simulink model "r2daq"  (R2012b)
settings: Solver=FixedStepDiscrete  SolverMode=SingleTasking  StartTime=0.0  StopTime=10.0  RelTol=1e-3
PreLoadFcn:
  | addpath(genpath('../lib/'));
model workspace (MAT data in the model file):
  pd_coeffbanks = 4
  pd_synthconf = 4
  pd_ctrl_reg = 4
  pd_ddc_2nd_stage = 64
  pd_status_reg = 4
  delay_time_pkt_vs_freq_pkt = 1536
  pd_to_status = 16
  pd_quantize = 16
undefined symbols (not defined in the file or in its folder): sfp
libraries: xbsIndex_r4 x1116, filters x8, r2daq_blocks x7, casper_library_misc x6, xps_library x3, synths x1, simulink x1
(part 1 of 14)
settings Model: Creator=ayoung  LastModifiedBy=ayoung
settings DebuggingCC: SigSpecEnsureSampleTimeMsg=none

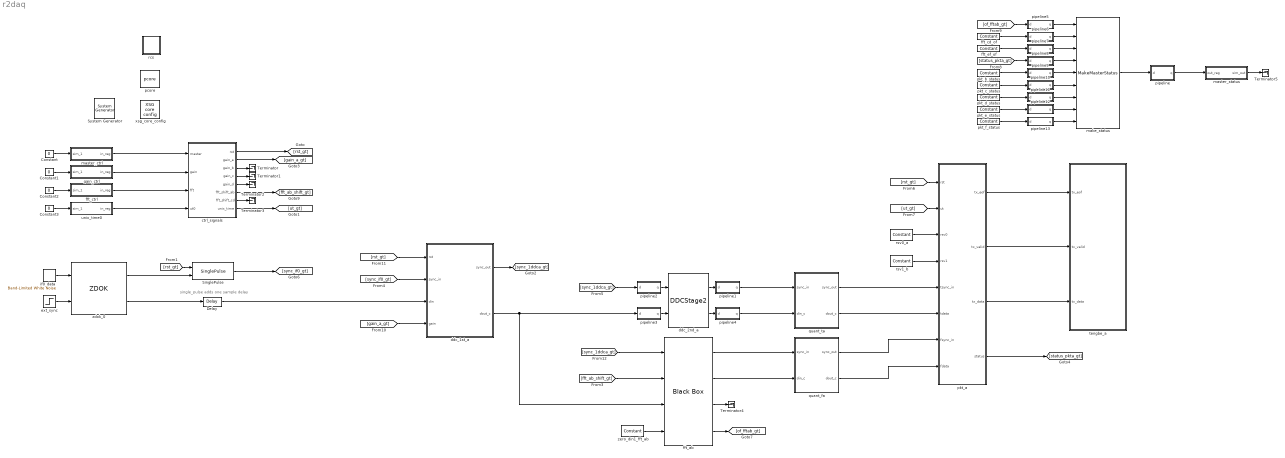
== system r2daq ==
  note: single_pulse adds one sample delay
  " System Generator" : xbsIndex_r4/ System Generator  Tag=genX  xilinxfamily=virtex6  part=xc6vsx475t  speed=-1  package=ff1759  synthesis_tool=XST  clock_wrapper=Clock Enables  directory=./r2daq/sysgen  proj_type=Project Navigator  Synth_file=XST Defaults  Impl_file=ISE Defaults  testbench=off  simulink_period=1  sysclk_period=5  dcm_input_clock_period=100  incr_netlist=off  trim_vbits=Everywhere in SubSystem  dbl_ovrd=According to Block Masks  core_generation=According to Block Masks  run_coregen=off  deprecated_control=off  eval_field=0  block_type=sysgen
  Constant{,1..3} (4 alike) : Constant  Value=0
  Delay : xbsIndex_r4/Delay  rst=off  infoeditControl=Selection of Reset will increase slice count due to use of real FFs and instead of SRLs  en=off  latency=1  dbl_ovrd=off  reg_retiming=off  block_type=delay
  SinglePulse : r2daq_blocks/SinglePulse
  Terminator{,1..5} (6 alike) : Terminator
  ctrl_signals : Subsystem
  ddc_1st_a : Subsystem
  ddc_2nd_a : r2daq_blocks/DDCStage2
  ext_sync : Step  SampleTime=0
  fft_ab : xbsIndex_r4/Black Box  init_code=fft_core_config  sim_method=Inactive  verbose=off  block_type=blackbox2
  fft_cd_of : xbsIndex_r4/Constant  const=0  gui_display_data_type=Boolean  arith_type=Boolean  n_bits=4  bin_pt=0  preci_type=Single  exp_width=8  frac_width=24  explicit_period=on  period=1  equ=P=C  opselect=C  inp2=PCIN>>17  opr=+  inp1=P  carry=CIN  dbl_ovrd=off  block_type=constant
  fft_ctrl : Subsystem  Tag=xps:sw_reg  AncestorBlock=xps_library/software_register  mask(swreg){mode=one value, io_dir=From Processor, io_delay=0, sample_period=1, names=reg, bitwidths=32, arith_types=0, bin_pts=0, sim_port=on, show_format=off}
      mask prompts: io_dir "I/O direction"; io_delay "I/O delay"; sample_period "Sample period"; names "Name:"; bitwidths "Bitwidth:"; arith_types "Type (ufix=0, fix=1, bool=2):"; bin_pts "Binary pt:"; sim_port "Provide sim input/output?"; show_format "Print format string?"
      mask init:
      | swreg_init(gcb)
      settings: AttributesFormatString=1input
      mask TypeOptions mode: one value | fields of equal size | fields of arbitrary size
      mask Callback mode: swreg_cb(gcb);
      mask TypeOptions io_dir: To Processor | From Processor
      mask Callback io_dir:
      | mask_enables = get_param(gcb, 'MaskEnables');
      | mask_names = get_param(gcb, 'MaskNames');
      | if strcmp(get_param(gcb, 'io_dir'), 'To Processor'),
      |     mask_enables{ismember(mask_names, 'sample_period')} = 'off';
      | else
      |     mask_enables{ismember(mask_names, 'sample_period')} = 'on';
      | end
      | set_param(gcb, 'MaskEnables', mask_enables);
      mask Callback bitwidths:
      | swreg_maskcheck(gcb);
      | % blk = gcb;
      | % mode = get_param(blk, 'mode');
      | % current_widths = eval(get_param(blk, 'bitwidths'));
      | % if (strcmp(mode, 'one value') || strcmp(mode, 'fields of equal size')) && (length(current_widths) > 1),
      | %     error('Only one width may be specified for this mode.');
      | % elseif strcmp(mode, 'fields of arbitrary size')
      | %     current_names = textscan(strtrim(strrep(strrep(get_param(blk, 'names'), ']', ''), '[', '')), '%s');
      | %     current_names = current_names{1};
      | %     numios = length(current_names);
      | %     if length(current_widths) ~= numios,
      | %         error('%d field names specified, but %d widths?', numios, length(current_widths));
      | %     end
      | % end
      | % total_width = 0;
      | % for ctr = 1 : length(current_widths),
      | %     total_width = total_width + current_widths(ctr);
      | % end
      | % if total_width > 32,
      | %     error('Total width must be 32 or less, set to %d.', total_width);
      | % end
      mask Callback arith_types:
      | [numios, ~, ~, ~, current_types] = swreg_maskcheck(gcb);
      | % blk = gcb;
      | % mode = get_param(blk, 'mode');
      | % current_types = eval(get_param(blk, 'arith_types'));
      | % numios = length(current_types);
      | % if (strcmp(mode, 'one value') || strcmp(mode, 'fields of equal size')) && (length(current_types) > 1),
      | %     error('Only one type may be specified for this mode.');
      | % elseif strcmp(mode, 'fields of arbitrary size')
      | %     current_names = textscan(strtrim(strrep(strrep(get_param(blk, 'names'), ']', ''), '[', '')), '%s');
      | %     current_names = current_names{1};
      | %     numios = length(current_names);
      | %     if length(current_types) ~= numios,
      | %         error('%d field names specified, but %d types?', numios, length(current_types));
      | %     end
      | % end
      | problem = 0;
      | for ctr = 1 : numios,
      |     t = current_types(ctr);
      |     if (t < 0) || (t > 2),
      |         problem = t;
      |         ctr = numios + 1;
      |     end
      | end
      | if problem ~= 0,
      |     error('Type cannot be %i, must be 0, 1 or 2.', problem);
      | end
      mask Callback bin_pts:
      | swreg_maskcheck(gcb);
      | % blk = gcb;
      | % mode = get_param(blk, 'mode');
      | % current_bins = eval(get_param(blk, 'bin_pts'));
      | % if (strcmp(mode, 'one value') || strcmp(mode, 'fields of equal size')) && (length(current_bins) > 1),
      | %     error('Only one binary pt may be specified for this mode.');
      | % elseif strcmp(mode, 'fields of arbitrary size')
      | %     current_names = textscan(strtrim(strrep(strrep(get_param(blk, 'names'), ']', ''), '[', '')), '%s');
      | %     current_names = current_names{1};
      | %     numios = length(current_names);
      | %     if length(current_bins) ~= numios,
      | %         error('%d field names specified, but %d binary pts?', numios, length(current_bins));
      | %     end
      | % end
  fft_ef_of : xbsIndex_r4/Constant  const=0  gui_display_data_type=Boolean  arith_type=Boolean  n_bits=4  bin_pt=0  preci_type=Single  exp_width=8  frac_width=24  explicit_period=on  period=1  equ=P=C  opselect=C  inp2=PCIN>>17  opr=+  inp1=P  carry=CIN  dbl_ovrd=off  block_type=constant
  gain_ctrl : Subsystem  Tag=xps:sw_reg  AncestorBlock=xps_library/software_register  mask(swreg){mode=one value, io_dir=From Processor, io_delay=0, sample_period=1, names=reg, bitwidths=32, arith_types=0, bin_pts=0, sim_port=on, show_format=off}
      mask prompts: io_dir "I/O direction"; io_delay "I/O delay"; sample_period "Sample period"; names "Name:"; bitwidths "Bitwidth:"; arith_types "Type (ufix=0, fix=1, bool=2):"; bin_pts "Binary pt:"; sim_port "Provide sim input/output?"; show_format "Print format string?"
      mask init:
      | swreg_init(gcb)
      settings: AttributesFormatString=1input
      mask TypeOptions mode: one value | fields of equal size | fields of arbitrary size
      mask Callback mode: swreg_cb(gcb);
      mask TypeOptions io_dir: To Processor | From Processor
      mask Callback io_dir:
      | mask_enables = get_param(gcb, 'MaskEnables');
      | mask_names = get_param(gcb, 'MaskNames');
      | if strcmp(get_param(gcb, 'io_dir'), 'To Processor'),
      |     mask_enables{ismember(mask_names, 'sample_period')} = 'off';
      | else
      |     mask_enables{ismember(mask_names, 'sample_period')} = 'on';
      | end
      | set_param(gcb, 'MaskEnables', mask_enables);
      mask Callback bitwidths:
      | swreg_maskcheck(gcb);
      | % blk = gcb;
      | % mode = get_param(blk, 'mode');
      | % current_widths = eval(get_param(blk, 'bitwidths'));
      | % if (strcmp(mode, 'one value') || strcmp(mode, 'fields of equal size')) && (length(current_widths) > 1),
      | %     error('Only one width may be specified for this mode.');
      | % elseif strcmp(mode, 'fields of arbitrary size')
      | %     current_names = textscan(strtrim(strrep(strrep(get_param(blk, 'names'), ']', ''), '[', '')), '%s');
      | %     current_names = current_names{1};
      | %     numios = length(current_names);
      | %     if length(current_widths) ~= numios,
      | %         error('%d field names specified, but %d widths?', numios, length(current_widths));
      | %     end
      | % end
      | % total_width = 0;
      | % for ctr = 1 : length(current_widths),
      | %     total_width = total_width + current_widths(ctr);
      | % end
      | % if total_width > 32,
      | %     error('Total width must be 32 or less, set to %d.', total_width);
      | % end
      mask Callback arith_types:
      | [numios, ~, ~, ~, current_types] = swreg_maskcheck(gcb);
      | % blk = gcb;
      | % mode = get_param(blk, 'mode');
      | % current_types = eval(get_param(blk, 'arith_types'));
      | % numios = length(current_types);
      | % if (strcmp(mode, 'one value') || strcmp(mode, 'fields of equal size')) && (length(current_types) > 1),
      | %     error('Only one type may be specified for this mode.');
      | % elseif strcmp(mode, 'fields of arbitrary size')
      | %     current_names = textscan(strtrim(strrep(strrep(get_param(blk, 'names'), ']', ''), '[', '')), '%s');
      | %     current_names = current_names{1};
      | %     numios = length(current_names);
      | %     if length(current_types) ~= numios,
      | %         error('%d field names specified, but %d types?', numios, length(current_types));
      | %     end
      | % end
      | problem = 0;
      | for ctr = 1 : numios,
      |     t = current_types(ctr);
      |     if (t < 0) || (t > 2),
      |         problem = t;
      |         ctr = numios + 1;
      |     end
      | end
      | if problem ~= 0,
      |     error('Type cannot be %i, must be 0, 1 or 2.', problem);
      | end
      mask Callback bin_pts:
      | swreg_maskcheck(gcb);
      | % blk = gcb;
      | % mode = get_param(blk, 'mode');
      | % current_bins = eval(get_param(blk, 'bin_pts'));
      | % if (strcmp(mode, 'one value') || strcmp(mode, 'fields of equal size')) && (length(current_bins) > 1),
      | %     error('Only one binary pt may be specified for this mode.');
      | % elseif strcmp(mode, 'fields of arbitrary size')
      | %     current_names = textscan(strtrim(strrep(strrep(get_param(blk, 'names'), ']', ''), '[', '')), '%s');
      | %     current_names = current_names{1};
      | %     numios = length(current_names);
      | %     if length(current_bins) ~= numios,
      | %         error('%d field names specified, but %d binary pts?', numios, length(current_bins));
      | %     end
      | % end
  if0_data : simulink/Sources/Band-Limited White Noise  Cov=[0.1]  Ts=0.1  seed=[23341]
  make_status : r2daq_blocks/MakeMasterStatus
  master_ctrl : Subsystem  Tag=xps:sw_reg  AncestorBlock=xps_library/software_register  mask(swreg){mode=one value, io_dir=From Processor, io_delay=0, sample_period=1, names=reg, bitwidths=32, arith_types=0, bin_pts=0, sim_port=on, show_format=off}
      mask prompts: io_dir "I/O direction"; io_delay "I/O delay"; sample_period "Sample period"; names "Name:"; bitwidths "Bitwidth:"; arith_types "Type (ufix=0, fix=1, bool=2):"; bin_pts "Binary pt:"; sim_port "Provide sim input/output?"; show_format "Print format string?"
      mask init:
      | swreg_init(gcb)
      settings: AttributesFormatString=1input
      mask TypeOptions mode: one value | fields of equal size | fields of arbitrary size
      mask Callback mode: swreg_cb(gcb);
      mask TypeOptions io_dir: To Processor | From Processor
      mask Callback io_dir:
      | mask_enables = get_param(gcb, 'MaskEnables');
      | mask_names = get_param(gcb, 'MaskNames');
      | if strcmp(get_param(gcb, 'io_dir'), 'To Processor'),
      |     mask_enables{ismember(mask_names, 'sample_period')} = 'off';
      | else
      |     mask_enables{ismember(mask_names, 'sample_period')} = 'on';
      | end
      | set_param(gcb, 'MaskEnables', mask_enables);
      mask Callback bitwidths:
      | swreg_maskcheck(gcb);
      | % blk = gcb;
      | % mode = get_param(blk, 'mode');
      | % current_widths = eval(get_param(blk, 'bitwidths'));
      | % if (strcmp(mode, 'one value') || strcmp(mode, 'fields of equal size')) && (length(current_widths) > 1),
      | %     error('Only one width may be specified for this mode.');
      | % elseif strcmp(mode, 'fields of arbitrary size')
      | %     current_names = textscan(strtrim(strrep(strrep(get_param(blk, 'names'), ']', ''), '[', '')), '%s');
      | %     current_names = current_names{1};
      | %     numios = length(current_names);
      | %     if length(current_widths) ~= numios,
      | %         error('%d field names specified, but %d widths?', numios, length(current_widths));
      | %     end
      | % end
      | % total_width = 0;
      | % for ctr = 1 : length(current_widths),
      | %     total_width = total_width + current_widths(ctr);
      | % end
      | % if total_width > 32,
      | %     error('Total width must be 32 or less, set to %d.', total_width);
      | % end
      mask Callback arith_types:
      | [numios, ~, ~, ~, current_types] = swreg_maskcheck(gcb);
      | % blk = gcb;
      | % mode = get_param(blk, 'mode');
      | % current_types = eval(get_param(blk, 'arith_types'));
      | % numios = length(current_types);
      | % if (strcmp(mode, 'one value') || strcmp(mode, 'fields of equal size')) && (length(current_types) > 1),
      | %     error('Only one type may be specified for this mode.');
      | % elseif strcmp(mode, 'fields of arbitrary size')
      | %     current_names = textscan(strtrim(strrep(strrep(get_param(blk, 'names'), ']', ''), '[', '')), '%s');
      | %     current_names = current_names{1};
      | %     numios = length(current_names);
      | %     if length(current_types) ~= numios,
      | %         error('%d field names specified, but %d types?', numios, length(current_types));
      | %     end
      | % end
      | problem = 0;
      | for ctr = 1 : numios,
      |     t = current_types(ctr);
      |     if (t < 0) || (t > 2),
      |         problem = t;
      |         ctr = numios + 1;
      |     end
      | end
      | if problem ~= 0,
      |     error('Type cannot be %i, must be 0, 1 or 2.', problem);
      | end
      mask Callback bin_pts:
      | swreg_maskcheck(gcb);
      | % blk = gcb;
      | % mode = get_param(blk, 'mode');
      | % current_bins = eval(get_param(blk, 'bin_pts'));
      | % if (strcmp(mode, 'one value') || strcmp(mode, 'fields of equal size')) && (length(current_bins) > 1),
      | %     error('Only one binary pt may be specified for this mode.');
      | % elseif strcmp(mode, 'fields of arbitrary size')
      | %     current_names = textscan(strtrim(strrep(strrep(get_param(blk, 'names'), ']', ''), '[', '')), '%s');
      | %     current_names = current_names{1};
      | %     numios = length(current_names);
      | %     if length(current_bins) ~= numios,
      | %         error('%d field names specified, but %d binary pts?', numios, length(current_bins));
      | %     end
      | % end
  master_status : Subsystem  Tag=xps:sw_reg  AncestorBlock=xps_library/software register  mask(swreg){mode=one value, io_dir=To Processor, io_delay=0, sample_period=1, names=reg, bitwidths=32, arith_types=0, bin_pts=0, sim_port=on, show_format=off}
      mask prompts: io_dir "I/O direction"; io_delay "I/O delay"; sample_period "Sample period"; names "Name:"; bitwidths "Bitwidth:"; arith_types "Type (ufix=0, fix=1, bool=2):"; bin_pts "Binary pt:"; sim_port "Provide sim input/output?"; show_format "Print format string?"
      mask init:
      | swreg_init(gcb)
      settings: AttributesFormatString=1output
      mask TypeOptions mode: one value | fields of equal size | fields of arbitrary size
      mask Callback mode: swreg_cb(gcb);
      mask TypeOptions io_dir: To Processor | From Processor
      mask Callback io_dir:
      | mask_enables = get_param(gcb, 'MaskEnables');
      | mask_names = get_param(gcb, 'MaskNames');
      | if strcmp(get_param(gcb, 'io_dir'), 'To Processor'),
      |     mask_enables{ismember(mask_names, 'sample_period')} = 'off';
      | else
      |     mask_enables{ismember(mask_names, 'sample_period')} = 'on';
      | end
      | set_param(gcb, 'MaskEnables', mask_enables);
      mask Callback bitwidths:
      | swreg_maskcheck(gcb);
      | % blk = gcb;
      | % mode = get_param(blk, 'mode');
      | % current_widths = eval(get_param(blk, 'bitwidths'));
      | % if (strcmp(mode, 'one value') || strcmp(mode, 'fields of equal size')) && (length(current_widths) > 1),
      | %     error('Only one width may be specified for this mode.');
      | % elseif strcmp(mode, 'fields of arbitrary size')
      | %     current_names = textscan(strtrim(strrep(strrep(get_param(blk, 'names'), ']', ''), '[', '')), '%s');
      | %     current_names = current_names{1};
      | %     numios = length(current_names);
      | %     if length(current_widths) ~= numios,
      | %         error('%d field names specified, but %d widths?', numios, length(current_widths));
      | %     end
      | % end
      | % total_width = 0;
      | % for ctr = 1 : length(current_widths),
      | %     total_width = total_width + current_widths(ctr);
      | % end
      | % if total_width > 32,
      | %     error('Total width must be 32 or less, set to %d.', total_width);
      | % end
      mask Callback arith_types:
      | [numios, ~, ~, ~, current_types] = swreg_maskcheck(gcb);
      | % blk = gcb;
      | % mode = get_param(blk, 'mode');
      | % current_types = eval(get_param(blk, 'arith_types'));
      | % numios = length(current_types);
      | % if (strcmp(mode, 'one value') || strcmp(mode, 'fields of equal size')) && (length(current_types) > 1),
      | %     error('Only one type may be specified for this mode.');
      | % elseif strcmp(mode, 'fields of arbitrary size')
      | %     current_names = textscan(strtrim(strrep(strrep(get_param(blk, 'names'), ']', ''), '[', '')), '%s');
      | %     current_names = current_names{1};
      | %     numios = length(current_names);
      | %     if length(current_types) ~= numios,
      | %         error('%d field names specified, but %d types?', numios, length(current_types));
      | %     end
      | % end
      | problem = 0;
      | for ctr = 1 : numios,
      |     t = current_types(ctr);
      |     if (t < 0) || (t > 2),
      |         problem = t;
      |         ctr = numios + 1;
      |     end
      | end
      | if problem ~= 0,
      |     error('Type cannot be %i, must be 0, 1 or 2.', problem);
      | end
      mask Callback bin_pts:
      | swreg_maskcheck(gcb);
      | % blk = gcb;
      | % mode = get_param(blk, 'mode');
      | % current_bins = eval(get_param(blk, 'bin_pts'));
      | % if (strcmp(mode, 'one value') || strcmp(mode, 'fields of equal size')) && (length(current_bins) > 1),
      | %     error('Only one binary pt may be specified for this mode.');
      | % elseif strcmp(mode, 'fields of arbitrary size')
      | %     current_names = textscan(strtrim(strrep(strrep(get_param(blk, 'names'), ']', ''), '[', '')), '%s');
      | %     current_names = current_names{1};
      | %     numios = length(current_names);
      | %     if length(current_bins) ~= numios,
      | %         error('%d field names specified, but %d binary pts?', numios, length(current_bins));
      | %     end
      | % end
  pcore : xps_library/pcore  Tag=xps:pcore  pcore_path=fft_core/fft_core.ngc
  pipeline : Subsystem  AncestorBlock=casper_library_delays/pipeline  mask(pipeline){latency=pd_status_reg}
      mask help:
      | An explicitly laid-out delay line to avoid mapping to SRL16s
      | for use in pipelining to help achieve timing closure.
      mask init:
      | pipeline_init(gcb,'latency',latency);
      settings: AttributesFormatString=Latency = %<latency>
      mask Display:
      | port_label('input', 1, 'd');
      | port_label('output', 1, 'q');
      | disp(['Z^-', num2str(latency)]);
  pipeline1 : Subsystem  AncestorBlock=casper_library_delays/pipeline  mask(pipeline){latency=pd_ddc_2nd_stage}
      mask help:
      | An explicitly laid-out delay line to avoid mapping to SRL16s
      | for use in pipelining to help achieve timing closure.
      mask init:
      | pipeline_init(gcb,'latency',latency);
      settings: AttributesFormatString=Latency = %<latency>
      mask Display:
      | port_label('input', 1, 'd');
      | port_label('output', 1, 'q');
      | disp(['Z^-', num2str(latency)]);
  pipeline10 : Subsystem  AncestorBlock=casper_library_delays/pipeline  mask(pipeline){latency=pd_to_status}
      mask help:
      | An explicitly laid-out delay line to avoid mapping to SRL16s
      | for use in pipelining to help achieve timing closure.
      mask init:
      | pipeline_init(gcb,'latency',latency);
      settings: AttributesFormatString=Latency = %<latency>
      mask Display:
      | port_label('input', 1, 'd');
      | port_label('output', 1, 'q');
      | disp(['Z^-', num2str(latency)]);
  pipeline11 : Subsystem  AncestorBlock=casper_library_delays/pipeline  mask(pipeline){latency=pd_to_status}
      mask help:
      | An explicitly laid-out delay line to avoid mapping to SRL16s
      | for use in pipelining to help achieve timing closure.
      mask init:
      | pipeline_init(gcb,'latency',latency);
      settings: AttributesFormatString=Latency = %<latency>
      mask Display:
      | port_label('input', 1, 'd');
      | port_label('output', 1, 'q');
      | disp(['Z^-', num2str(latency)]);
  pipeline12 : Subsystem  AncestorBlock=casper_library_delays/pipeline  mask(pipeline){latency=pd_to_status}
      mask help:
      | An explicitly laid-out delay line to avoid mapping to SRL16s
      | for use in pipelining to help achieve timing closure.
      mask init:
      | pipeline_init(gcb,'latency',latency);
      settings: AttributesFormatString=Latency = %<latency>
      mask Display:
      | port_label('input', 1, 'd');
      | port_label('output', 1, 'q');
      | disp(['Z^-', num2str(latency)]);
  pipeline13 : Subsystem  AncestorBlock=casper_library_delays/pipeline  mask(pipeline){latency=pd_to_status}
      mask help:
      | An explicitly laid-out delay line to avoid mapping to SRL16s
      | for use in pipelining to help achieve timing closure.
      mask init:
      | pipeline_init(gcb,'latency',latency);
      settings: AttributesFormatString=Latency = %<latency>
      mask Display:
      | port_label('input', 1, 'd');
      | port_label('output', 1, 'q');
      | disp(['Z^-', num2str(latency)]);
  pipeline2 : Subsystem  AncestorBlock=casper_library_delays/pipeline  mask(pipeline){latency=pd_ddc_2nd_stage}
      mask help:
      | An explicitly laid-out delay line to avoid mapping to SRL16s
      | for use in pipelining to help achieve timing closure.
      mask init:
      | pipeline_init(gcb,'latency',latency);
      settings: AttributesFormatString=Latency = %<latency>
      mask Display:
      | port_label('input', 1, 'd');
      | port_label('output', 1, 'q');
      | disp(['Z^-', num2str(latency)]);
  pipeline3 : Subsystem  AncestorBlock=casper_library_delays/pipeline  mask(pipeline){latency=pd_ddc_2nd_stage}
      mask help:
      | An explicitly laid-out delay line to avoid mapping to SRL16s
      | for use in pipelining to help achieve timing closure.
      mask init:
      | pipeline_init(gcb,'latency',latency);
      settings: AttributesFormatString=Latency = %<latency>
      mask Display:
      | port_label('input', 1, 'd');
      | port_label('output', 1, 'q');
      | disp(['Z^-', num2str(latency)]);
  pipeline4 : Subsystem  AncestorBlock=casper_library_delays/pipeline  mask(pipeline){latency=pd_ddc_2nd_stage}
      mask help:
      | An explicitly laid-out delay line to avoid mapping to SRL16s
      | for use in pipelining to help achieve timing closure.
      mask init:
      | pipeline_init(gcb,'latency',latency);
      settings: AttributesFormatString=Latency = %<latency>
      mask Display:
      | port_label('input', 1, 'd');
      | port_label('output', 1, 'q');
      | disp(['Z^-', num2str(latency)]);
  pipeline5 : Subsystem  AncestorBlock=casper_library_delays/pipeline  mask(pipeline){latency=pd_to_status}
      mask help:
      | An explicitly laid-out delay line to avoid mapping to SRL16s
      | for use in pipelining to help achieve timing closure.
      mask init:
      | pipeline_init(gcb,'latency',latency);
      settings: AttributesFormatString=Latency = %<latency>
      mask Display:
      | port_label('input', 1, 'd');
      | port_label('output', 1, 'q');
      | disp(['Z^-', num2str(latency)]);
  pipeline6 : Subsystem  AncestorBlock=casper_library_delays/pipeline  mask(pipeline){latency=pd_to_status}
      mask help:
      | An explicitly laid-out delay line to avoid mapping to SRL16s
      | for use in pipelining to help achieve timing closure.
      mask init:
      | pipeline_init(gcb,'latency',latency);
      settings: AttributesFormatString=Latency = %<latency>
      mask Display:
      | port_label('input', 1, 'd');
      | port_label('output', 1, 'q');
      | disp(['Z^-', num2str(latency)]);
  pipeline7 : Subsystem  AncestorBlock=casper_library_delays/pipeline  mask(pipeline){latency=pd_to_status}
      mask help:
      | An explicitly laid-out delay line to avoid mapping to SRL16s
      | for use in pipelining to help achieve timing closure.
      mask init:
      | pipeline_init(gcb,'latency',latency);
      settings: AttributesFormatString=Latency = %<latency>
      mask Display:
      | port_label('input', 1, 'd');
      | port_label('output', 1, 'q');
      | disp(['Z^-', num2str(latency)]);
  pipeline8 : Subsystem  AncestorBlock=casper_library_delays/pipeline  mask(pipeline){latency=pd_to_status}
      mask help:
      | An explicitly laid-out delay line to avoid mapping to SRL16s
      | for use in pipelining to help achieve timing closure.
      mask init:
      | pipeline_init(gcb,'latency',latency);
      settings: AttributesFormatString=Latency = %<latency>
      mask Display:
      | port_label('input', 1, 'd');
      | port_label('output', 1, 'q');
      | disp(['Z^-', num2str(latency)]);
  pipeline9 : Subsystem  AncestorBlock=casper_library_delays/pipeline  mask(pipeline){latency=pd_to_status}
      mask help:
      | An explicitly laid-out delay line to avoid mapping to SRL16s
      | for use in pipelining to help achieve timing closure.
      mask init:
      | pipeline_init(gcb,'latency',latency);
      settings: AttributesFormatString=Latency = %<latency>
      mask Display:
      | port_label('input', 1, 'd');
      | port_label('output', 1, 'q');
      | disp(['Z^-', num2str(latency)]);
  pkt_a : Subsystem  AncestorBlock=r2daq_blocks/Packetizer  mask(Packetizer){N_fft=8192, frames_per_batch=390625, IF_ID=0, Digital_ID=0, pd_in=pd_ctrl_reg, pd_tvf=delay_time_pkt_vs_freq_pkt}
      mask prompts: N_fft "FFT-size"; frames_per_batch "Frames in batch"; IF_ID "IF ID (6-bit)"; Digital_ID "Digital ID (6-bit)"; pd_in "Pipeline delay registers"; pd_tvf "Time packet delay relative to frequency packet"
      mask help:
      | Packetizes simultaneous time- and frequency-domain data for transmission using a 10GbE core.
      |
      | An asynchronous reset port is available as rst.
      |
      | Complex-valued frequency-domain data is supplied as UFix_16_0 to fdata. A single pulse on fsync_in indicates that the first sample of valid data will appear at fdata on the next clock cycle. Only one such pulse should be given per reset. The same applies to tdata and tsync_in.
      |
      | Current unix-time can be supplied as a UFix_32_0 to port ut.
      |
      | 64bit-wide header data can be supplied to each rsv0 and rsv1. Note that b63 (msb) of rsv1 is over-written internally.
      |
      | Signals to drive a 10GbE core are directly available in tx_eof, tx_valid, and tx_data.
      |
      | Empty and full signals of internal FIFO's used to buffer time- and frequency-domain data are available in ffifo_empty, ffifo_full, tfifo_empty and tfifo_full.
      mask init:
      | pd_inst = {...
      |     [gcb '/pd_ud0'],...
      |     [gcb '/pd_ud1']};
      | pd_in = get_param(gcb,'pd_in');
      | for ii=1:numel(pd_inst)
      |     set_param(pd_inst{ii},'latency',pd_in);
      | end
      | pd_inst = [gcb '/pd_dtf'];
      | %pd_tvf = get_param(gcb,'pd_tvf');
      | %set_param(pd_inst,'latency',pd_tvf);
      | pd_tvf_delay = 4;
      | set_param([gcb '/data_per_frame'],'const',num2str(N_fft-1));
      | set_param([gcb '/fpb_const'],'const',num2str(frames_per_batch));
      | set_param([gcb '/pd_dtf_pre'],'latency',num2str(pd_tvf_delay));
      | set_param([gcb '/delay_neg_edge'],'latency',num2str(pd_tvf-2*pd_tvf_delay));
      | set_param([gcb '/pd_dtf_post'],'latency',num2str(pd_tvf_delay));
  pkt_b_status : xbsIndex_r4/Constant  const=0  gui_display_data_type=Fixed-point  arith_type=Unsigned  n_bits=4  bin_pt=0  preci_type=Single  exp_width=8  frac_width=24  explicit_period=on  period=1  equ=P=C  opselect=C  inp2=PCIN>>17  opr=+  inp1=P  carry=CIN  dbl_ovrd=off  block_type=constant
  pkt_c_status : xbsIndex_r4/Constant  const=0  gui_display_data_type=Fixed-point  arith_type=Unsigned  n_bits=4  bin_pt=0  preci_type=Single  exp_width=8  frac_width=24  explicit_period=on  period=1  equ=P=C  opselect=C  inp2=PCIN>>17  opr=+  inp1=P  carry=CIN  dbl_ovrd=off  block_type=constant
  pkt_d_status : xbsIndex_r4/Constant  const=0  gui_display_data_type=Fixed-point  arith_type=Unsigned  n_bits=4  bin_pt=0  preci_type=Single  exp_width=8  frac_width=24  explicit_period=on  period=1  equ=P=C  opselect=C  inp2=PCIN>>17  opr=+  inp1=P  carry=CIN  dbl_ovrd=off  block_type=constant
  pkt_e_status : xbsIndex_r4/Constant  const=0  gui_display_data_type=Fixed-point  arith_type=Unsigned  n_bits=4  bin_pt=0  preci_type=Single  exp_width=8  frac_width=24  explicit_period=on  period=1  equ=P=C  opselect=C  inp2=PCIN>>17  opr=+  inp1=P  carry=CIN  dbl_ovrd=off  block_type=constant
  pkt_f_status : xbsIndex_r4/Constant  const=0  gui_display_data_type=Fixed-point  arith_type=Unsigned  n_bits=4  bin_pt=0  preci_type=Single  exp_width=8  frac_width=24  explicit_period=on  period=1  equ=P=C  opselect=C  inp2=PCIN>>17  opr=+  inp1=P  carry=CIN  dbl_ovrd=off  block_type=constant
  quant_fa : Subsystem  AncestorBlock=r2daq_blocks/Quantize8bit  mask{pd_io=pd_quantize}
      mask prompts: pd_io "Pipeline delay"
      mask init:
      | pd_inst = {...
      |     [gcb '/pd_sync'],...
      |     [gcb '/pd_data']};
      | pd_io = get_param(gcb,'pd_io');
      | for ii=1:numel(pd_inst)
      |     set_param(pd_inst{ii},'latency',pd_io);
      | end
  quant_ta : Subsystem  AncestorBlock=r2daq_blocks/Quantize8bit  mask{pd_io=pd_quantize}
      mask prompts: pd_io "Pipeline delay"
      mask init:
      | pd_inst = {...
      |     [gcb '/pd_sync'],...
      |     [gcb '/pd_data']};
      | pd_io = get_param(gcb,'pd_io');
      | for ii=1:numel(pd_inst)
      |     set_param(pd_inst{ii},'latency',pd_io);
      | end
  rcs : Subsystem  AncestorBlock=casper_library_misc/rcs  mask(rcs){app_src=git, lib_src=git, user_val=0}
      mask prompts: app_src "Application revision info to capture"; lib_src "CASPER libraries revision info to capture"; user_val "User specified value"
      mask help:
      | Embeds revision control information for the user design and libraries.
      | On failure to locate specified revision information, falls back to
      | timestamps (current time for libraries).
      | A user specified value is also stored.
      mask init:
      | rcs_init(gcb, ...
      |     'app_src', app_src, ...
      |     'lib_src', lib_src);
      mask TypeOptions app_src: timestamp | git | svn
      mask TypeOptions lib_src: timestamp | git | svn
  rsv0_a : xbsIndex_r4/Constant  const=0  gui_display_data_type=Fixed-point  arith_type=Unsigned  n_bits=64  bin_pt=0  preci_type=Single  exp_width=8  frac_width=24  explicit_period=on  period=1  equ=P=C  opselect=C  inp2=PCIN>>17  opr=+  inp1=P  carry=CIN  dbl_ovrd=off  block_type=constant
  rsv1_b : xbsIndex_r4/Constant  const=0  gui_display_data_type=Fixed-point  arith_type=Unsigned  n_bits=64  bin_pt=0  preci_type=Single  exp_width=8  frac_width=24  explicit_period=on  period=1  equ=P=C  opselect=C  inp2=PCIN>>17  opr=+  inp1=P  carry=CIN  dbl_ovrd=off  block_type=constant
  tengbe_a : Subsystem  AncestorBlock=r2daq_blocks/TenGbEWrap  mask(TenGbEWrap){pd_in=pd_ctrl_reg, pd_out=pd_status_reg}
      mask prompts: pd_in "Registers in pipeline delay"; pd_out "Registers out pipeline delay"
      mask help:
      | Wrap 10GbE core and supplies control and status registers internally.
      |
      | Pipeline delay to and from registers are configurable.
      mask init:
      | pd_inst = {...
      |     [gcb '/pd_ctrl'],...
      |     [gcb '/pd_port'],...
      |     [gcb '/pd_ip']};
      | pd_in = get_param(gcb,'pd_in');
      | for ii=1:numel(pd_inst)
      |     set_param(pd_inst{ii},'latency',pd_in);
      | end
      | pd_inst = {...
      |     [gcb '/pd_status']};
      | pd_out = get_param(gcb,'pd_out');
      | for ii=1:numel(pd_inst)
      |     set_param(pd_inst{ii},'latency',pd_out);
      | end
  unix_time0 : Subsystem  Tag=xps:sw_reg  AncestorBlock=xps_library/software_register  mask(swreg){mode=one value, io_dir=From Processor, io_delay=0, sample_period=1, names=reg, bitwidths=32, arith_types=0, bin_pts=0, sim_port=on, show_format=off}
      mask prompts: io_dir "I/O direction"; io_delay "I/O delay"; sample_period "Sample period"; names "Name:"; bitwidths "Bitwidth:"; arith_types "Type (ufix=0, fix=1, bool=2):"; bin_pts "Binary pt:"; sim_port "Provide sim input/output?"; show_format "Print format string?"
      mask init:
      | swreg_init(gcb)
      settings: AttributesFormatString=1input
      mask TypeOptions mode: one value | fields of equal size | fields of arbitrary size
      mask Callback mode: swreg_cb(gcb);
      mask TypeOptions io_dir: To Processor | From Processor
      mask Callback io_dir:
      | mask_enables = get_param(gcb, 'MaskEnables');
      | mask_names = get_param(gcb, 'MaskNames');
      | if strcmp(get_param(gcb, 'io_dir'), 'To Processor'),
      |     mask_enables{ismember(mask_names, 'sample_period')} = 'off';
      | else
      |     mask_enables{ismember(mask_names, 'sample_period')} = 'on';
      | end
      | set_param(gcb, 'MaskEnables', mask_enables);
      mask Callback bitwidths:
      | swreg_maskcheck(gcb);
      | % blk = gcb;
      | % mode = get_param(blk, 'mode');
      | % current_widths = eval(get_param(blk, 'bitwidths'));
      | % if (strcmp(mode, 'one value') || strcmp(mode, 'fields of equal size')) && (length(current_widths) > 1),
      | %     error('Only one width may be specified for this mode.');
      | % elseif strcmp(mode, 'fields of arbitrary size')
      | %     current_names = textscan(strtrim(strrep(strrep(get_param(blk, 'names'), ']', ''), '[', '')), '%s');
      | %     current_names = current_names{1};
      | %     numios = length(current_names);
      | %     if length(current_widths) ~= numios,
      | %         error('%d field names specified, but %d widths?', numios, length(current_widths));
      | %     end
      | % end
      | % total_width = 0;
      | % for ctr = 1 : length(current_widths),
      | %     total_width = total_width + current_widths(ctr);
      | % end
      | % if total_width > 32,
      | %     error('Total width must be 32 or less, set to %d.', total_width);
      | % end
      mask Callback arith_types:
      | [numios, ~, ~, ~, current_types] = swreg_maskcheck(gcb);
      | % blk = gcb;
      | % mode = get_param(blk, 'mode');
      | % current_types = eval(get_param(blk, 'arith_types'));
      | % numios = length(current_types);
      | % if (strcmp(mode, 'one value') || strcmp(mode, 'fields of equal size')) && (length(current_types) > 1),
      | %     error('Only one type may be specified for this mode.');
      | % elseif strcmp(mode, 'fields of arbitrary size')
      | %     current_names = textscan(strtrim(strrep(strrep(get_param(blk, 'names'), ']', ''), '[', '')), '%s');
      | %     current_names = current_names{1};
      | %     numios = length(current_names);
      | %     if length(current_types) ~= numios,
      | %         error('%d field names specified, but %d types?', numios, length(current_types));
      | %     end
      | % end
      | problem = 0;
      | for ctr = 1 : numios,
      |     t = current_types(ctr);
      |     if (t < 0) || (t > 2),
      |         problem = t;
      |         ctr = numios + 1;
      |     end
      | end
      | if problem ~= 0,
      |     error('Type cannot be %i, must be 0, 1 or 2.', problem);
      | end
      mask Callback bin_pts:
      | swreg_maskcheck(gcb);
      | % blk = gcb;
      | % mode = get_param(blk, 'mode');
      | % current_bins = eval(get_param(blk, 'bin_pts'));
      | % if (strcmp(mode, 'one value') || strcmp(mode, 'fields of equal size')) && (length(current_bins) > 1),
      | %     error('Only one binary pt may be specified for this mode.');
      | % elseif strcmp(mode, 'fields of arbitrary size')
      | %     current_names = textscan(strtrim(strrep(strrep(get_param(blk, 'names'), ']', ''), '[', '')), '%s');
      | %     current_names = current_names{1};
      | %     numios = length(current_names);
      | %     if length(current_bins) ~= numios,
      | %         error('%d field names specified, but %d binary pts?', numios, length(current_bins));
      | %     end
      | % end
  xsg_core_config : xps_library/XSG core config  Tag=xps:xsg  hw_sys=ROACH2:sx475t  clk_src=adc0_clk  ROACH_clk_src=sys_clk  ROACH2_clk_src=adc0_clk  MKDIG_clk_src=sys_clk  clk_rate=200  sample_period=1  synthesis_tool=XST
  zdok_0 : r2daq_blocks/ZDOK  zdok_slot=ZDOK 0  freq_nyq=1600
      link override asiaa_adc5g: adc_brd=ZDOK 0  adc_bit_width=8  adc_clk_rate=1600
      link override asiaa_adc5g/a0: Port=1
      link override asiaa_adc5g/a1: Port=2
      link override asiaa_adc5g/a10: Port=11
      link override asiaa_adc5g/a11: Port=12
      link override asiaa_adc5g/a12: Port=13
      link override asiaa_adc5g/a13: Port=14
      link override asiaa_adc5g/a14: Port=15
      link override asiaa_adc5g/a15: Port=16
      link override asiaa_adc5g/a2: Port=3
      link override asiaa_adc5g/a3: Port=4
      link override asiaa_adc5g/a4: Port=5
      link override asiaa_adc5g/a5: Port=6
      link override asiaa_adc5g/a6: Port=7
      link override asiaa_adc5g/a7: Port=8
      link override asiaa_adc5g/a8: Port=9
      link override asiaa_adc5g/a9: Port=10
      link override asiaa_adc5g/bias_a: Bias=128
      link override asiaa_adc5g/delay_a0: DelayLength=2
      link override asiaa_adc5g/delay_a1: DelayLength=1
      link override asiaa_adc5g/delay_a10: DelayLength=1
      link override asiaa_adc5g/delay_a11: DelayLength=1
      link override asiaa_adc5g/delay_a12: DelayLength=1
      link override asiaa_adc5g/delay_a13: DelayLength=1
      link override asiaa_adc5g/delay_a14: DelayLength=1
      link override asiaa_adc5g/delay_a15: DelayLength=1
      link override asiaa_adc5g/delay_a2: DelayLength=1
      link override asiaa_adc5g/delay_a3: DelayLength=1
      link override asiaa_adc5g/delay_a4: DelayLength=1
      link override asiaa_adc5g/delay_a5: DelayLength=1
      link override asiaa_adc5g/delay_a6: DelayLength=1
      link override asiaa_adc5g/delay_a7: DelayLength=1
      link override asiaa_adc5g/delay_a8: DelayLength=1
      link override asiaa_adc5g/delay_a9: DelayLength=1
      link override asiaa_adc5g/downsample_a0: N=16  phase=0  RateOptions=Allow multirate processing  ic=0
      link override asiaa_adc5g/downsample_a1: N=16  phase=1  RateOptions=Allow multirate processing  ic=0
      link override asiaa_adc5g/downsample_a10: N=16  phase=10  RateOptions=Allow multirate processing  ic=0
      link override asiaa_adc5g/downsample_a11: N=16  phase=11  RateOptions=Allow multirate processing  ic=0
      link override asiaa_adc5g/downsample_a12: N=16  phase=12  RateOptions=Allow multirate processing  ic=0
      link override asiaa_adc5g/downsample_a13: N=16  phase=13  RateOptions=Allow multirate processing  ic=0
      link override asiaa_adc5g/downsample_a14: N=16  phase=14  RateOptions=Allow multirate processing  ic=0
      link override asiaa_adc5g/downsample_a15: N=16  phase=15  RateOptions=Allow multirate processing  ic=0
      link override asiaa_adc5g/downsample_a2: N=16  phase=2  RateOptions=Allow multirate processing  ic=0
      link override asiaa_adc5g/downsample_a3: N=16  phase=3  RateOptions=Allow multirate processing  ic=0
      link override asiaa_adc5g/downsample_a4: N=16  phase=4  RateOptions=Allow multirate processing  ic=0
      link override asiaa_adc5g/downsample_a5: N=16  phase=5  RateOptions=Allow multirate processing  ic=0
      link override asiaa_adc5g/downsample_a6: N=16  phase=6  RateOptions=Allow multirate processing  ic=0
      link override asiaa_adc5g/downsample_a7: N=16  phase=7  RateOptions=Allow multirate processing  ic=0
      link override asiaa_adc5g/downsample_a8: N=16  phase=8  RateOptions=Allow multirate processing  ic=0
      link override asiaa_adc5g/downsample_a9: N=16  phase=9  RateOptions=Allow multirate processing  ic=0
      link override asiaa_adc5g/gain_a: Gain=128
      link override asiaa_adc5g/sim_a: Port=1
      link override asiaa_adc5g/sim_sync: Port=2
      link override asiaa_adc5g/simulink_need_slupdate_PID_Controller_with_Approximate_Derivative_sync: arith_type=Boolean
      link override asiaa_adc5g/simulink_need_slupdate_PID_Controller_with_Approximate_Derivative_user_data_i0: arith_type=Unsigned  n_bits=8  bin_pt=0  quantization=Truncate  overflow=Wrap
      link override asiaa_adc5g/simulink_need_slupdate_PID_Controller_with_Approximate_Derivative_user_data_i1: arith_type=Unsigned  n_bits=8  bin_pt=0  quantization=Truncate  overflow=Wrap
      link override asiaa_adc5g/simulink_need_slupdate_PID_Controller_with_Approximate_Derivative_user_data_i2: arith_type=Unsigned  n_bits=8  bin_pt=0  quantization=Truncate  overflow=Wrap
      link override asiaa_adc5g/simulink_need_slupdate_PID_Controller_with_Approximate_Derivative_user_data_i3: arith_type=Unsigned  n_bits=8  bin_pt=0  quantization=Truncate  overflow=Wrap
      link override asiaa_adc5g/simulink_need_slupdate_PID_Controller_with_Approximate_Derivative_user_data_i4: arith_type=Unsigned  n_bits=8  bin_pt=0  quantization=Truncate  overflow=Wrap
      link override asiaa_adc5g/simulink_need_slupdate_PID_Controller_with_Approximate_Derivative_user_data_i5: arith_type=Unsigned  n_bits=8  bin_pt=0  quantization=Truncate  overflow=Wrap
      link override asiaa_adc5g/simulink_need_slupdate_PID_Controller_with_Approximate_Derivative_user_data_i6: arith_type=Unsigned  n_bits=8  bin_pt=0  quantization=Truncate  overflow=Wrap
      link override asiaa_adc5g/simulink_need_slupdate_PID_Controller_with_Approximate_Derivative_user_data_i7: arith_type=Unsigned  n_bits=8  bin_pt=0  quantization=Truncate  overflow=Wrap
      link override asiaa_adc5g/simulink_need_slupdate_PID_Controller_with_Approximate_Derivative_user_data_q0: arith_type=Unsigned  n_bits=8  bin_pt=0  quantization=Truncate  overflow=Wrap
      link override asiaa_adc5g/simulink_need_slupdate_PID_Controller_with_Approximate_Derivative_user_data_q1: arith_type=Unsigned  n_bits=8  bin_pt=0  quantization=Truncate  overflow=Wrap
      link override asiaa_adc5g/simulink_need_slupdate_PID_Controller_with_Approximate_Derivative_user_data_q2: arith_type=Unsigned  n_bits=8  bin_pt=0  quantization=Truncate  overflow=Wrap
      link override asiaa_adc5g/simulink_need_slupdate_PID_Controller_with_Approximate_Derivative_user_data_q3: arith_type=Unsigned  n_bits=8  bin_pt=0  quantization=Truncate  overflow=Wrap
      link override asiaa_adc5g/simulink_need_slupdate_PID_Controller_with_Approximate_Derivative_user_data_q4: arith_type=Unsigned  n_bits=8  bin_pt=0  quantization=Truncate  overflow=Wrap
      link override asiaa_adc5g/simulink_need_slupdate_PID_Controller_with_Approximate_Derivative_user_data_q5: arith_type=Unsigned  n_bits=8  bin_pt=0  quantization=Truncate  overflow=Wrap
      link override asiaa_adc5g/simulink_need_slupdate_PID_Controller_with_Approximate_Derivative_user_data_q6: arith_type=Unsigned  n_bits=8  bin_pt=0  quantization=Truncate  overflow=Wrap
      link override asiaa_adc5g/simulink_need_slupdate_PID_Controller_with_Approximate_Derivative_user_data_q7: arith_type=Unsigned  n_bits=8  bin_pt=0  quantization=Truncate  overflow=Wrap
      link override asiaa_adc5g/sync_out: Port=17
  zero_din1_fft_ab : xbsIndex_r4/Constant  const=0  gui_display_data_type=Fixed-point  arith_type=Unsigned  n_bits=50  bin_pt=0  preci_type=Single  exp_width=8  frac_width=24  explicit_period=on  period=1  equ=P=C  opselect=C  inp2=PCIN>>17  opr=+  inp1=P  carry=CIN  dbl_ovrd=off  block_type=constant
  wires:
  zdok_0/2 -> Delay/1
  [rst_gt] -> SinglePulse/1
  zdok_0/1 -> SinglePulse/2
  if0_data/1 -> zdok_0/1
  ext_sync/1 -> zdok_0/2
  [gain_a_gt] -> ddc_1st_a/4(gain)
  master_ctrl/1(in_reg) -> ctrl_signals/1(master)
  gain_ctrl/1(in_reg) -> ctrl_signals/2(gain)
  fft_ctrl/1(in_reg) -> ctrl_signals/3(fft)
  unix_time0/1(in_reg) -> ctrl_signals/4(ut0)
  ctrl_signals/1(rst) -> [rst_gt]
  ctrl_signals/2(gain_a) -> [gain_a_gt]
  ctrl_signals/6(fft_shift_ab) -> [fft_ab_shift_gt]
  SinglePulse/1 -> [sync_if0_gt]
  ctrl_signals/3(gain_b) -> Terminator/1
  ctrl_signals/4(gain_c) -> Terminator1/1
  ctrl_signals/5(gain_d) -> Terminator2/1
  ctrl_signals/7(fft_shift_cd) -> Terminator3/1
  ctrl_signals/8(unix_time) -> [ut_gt]
  Delay/1 -> ddc_1st_a/3(din)
  [sync_if0_gt] -> ddc_1st_a/2(sync_in)
  [rst_gt] -> ddc_1st_a/1(rst)
  ddc_2nd_a/1 -> pipeline1/1(d)
  ddc_2nd_a/2 -> pipeline4/1(d)
  pipeline2/1(q) -> ddc_2nd_a/1
  pipeline3/1(q) -> ddc_2nd_a/2
  ddc_1st_a/2(dout_c) -> fft_ab/3, pipeline3/1(d)
  ddc_1st_a/1(sync_out) -> [sync_1ddca_gt]
  [sync_1ddca_gt] -> pipeline2/1(d)
  pipeline1/1(q) -> quant_ta/1(sync_in)
  pipeline4/1(q) -> quant_ta/2(din_c)
  [rst_gt] -> pkt_a/1(rst)
  [ut_gt] -> pkt_a/2(ut)
  quant_ta/1(sync_out) -> pkt_a/5(tsync_in)
  quant_ta/2(dout_c) -> pkt_a/6(tdata)
  pkt_a/1(tx_eof) -> tengbe_a/1(tx_eof)
  pkt_a/2(tx_valid) -> tengbe_a/2(tx_valid)
  pkt_a/3(tx_data) -> tengbe_a/3(tx_data)
  pkt_a/4(status) -> [status_pkta_gt]
  rsv1_b/1 -> pkt_a/4(rsv1)
  rsv0_a/1 -> pkt_a/3(rsv0)
  make_status/1 -> pipeline/1(d)
  pipeline/1(q) -> master_status/1(out_reg)
  [sync_1ddca_gt] -> fft_ab/1
  [fft_ab_shift_gt] -> fft_ab/2
  fft_ab/2 -> quant_fa/2(din_c)
  quant_fa/1(sync_out) -> pkt_a/7(fsync_in)
  quant_fa/2(dout_c) -> pkt_a/8(fdata)
  fft_ab/1 -> quant_fa/1(sync_in)
  fft_ab/3 -> Terminator4/1
  fft_ab/4 -> [of_fftab_gt]
  zero_din1_fft_ab/1 -> fft_ab/4
  [of_fftab_gt] -> pipeline5/1(d)
  fft_cd_of/1 -> pipeline6/1(d)
  fft_ef_of/1 -> pipeline7/1(d)
  [status_pkta_gt] -> pipeline8/1(d)
  pkt_b_status/1 -> pipeline9/1(d)
  pkt_c_status/1 -> pipeline10/1(d)
  pkt_d_status/1 -> pipeline11/1(d)
  pkt_e_status/1 -> pipeline12/1(d)
  pkt_f_status/1 -> pipeline13/1(d)
  pipeline6/1(q) -> make_status/2
  pipeline11/1(q) -> make_status/7
  pipeline7/1(q) -> make_status/3
  pipeline9/1(q) -> make_status/5
  pipeline13/1(q) -> make_status/9
  pipeline8/1(q) -> make_status/4
  pipeline10/1(q) -> make_status/6
  pipeline12/1(q) -> make_status/8
  pipeline5/1(q) -> make_status/1
  Constant/1 -> master_ctrl/1(sim_1)
  Constant1/1 -> gain_ctrl/1(sim_1)
  Constant2/1 -> fft_ctrl/1(sim_1)
  Constant3/1 -> unix_time0/1(sim_1)
  master_status/1(sim_out) -> Terminator5/1
